simulink model "arducopter"  (R2021a)
settings: Solver=FixedStepAuto  StartTime=0.0  StopTime=sim.param.timeEnd  FixedStep=sim.param.dt  RelTol=1e-3
undefined symbols (not defined in the file or in its folder): DiscIntNeverNeededParam, sim
libraries: simulink x34, slident x4, vrlib x1
(part 3 of 8)

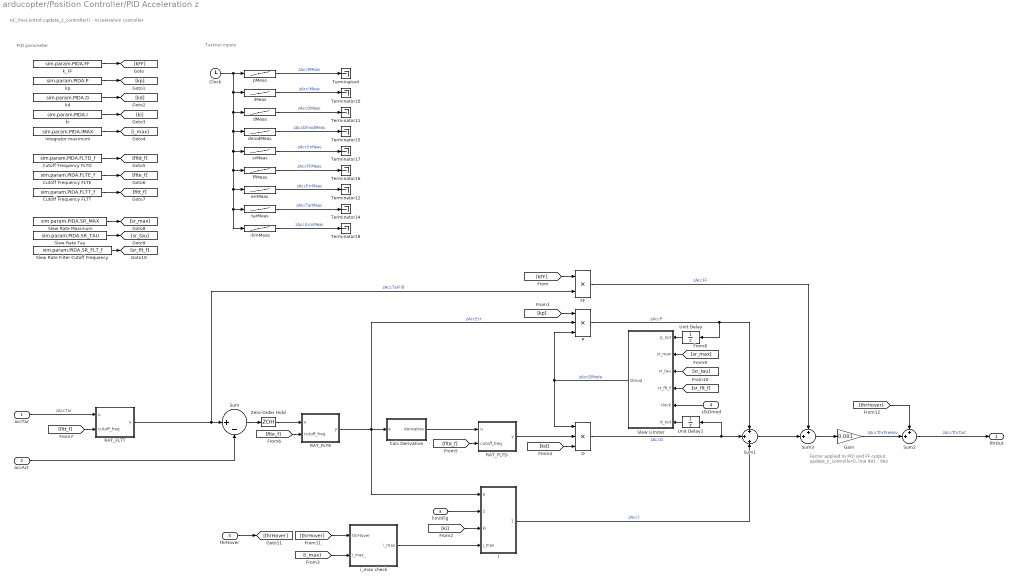
== system arducopter/Position Controller/PID Acceleration z ==
  note: Factor applied to PID and FF output.
      | update_z_controller(), line 991 - 992
  note: AC_PosControl::update_z_controller() - Acceleration controller
  note: PID parameter
  note: Testrun inputs
  accTar : Inport
  accAct : Inport  Port=2
  limitFlg : Inport  Port=3
  clkDmod : Inport  Port=4
  thrHover : Inport  Port=5
  Calc Derivative : Subsystem
  Clock : Clock
  Cutoff Frequency FLTD : Constant  Value=sim.param.PIDA.FLTD_f
  Cutoff Frequency FLTE : Constant  Value=sim.param.PIDA.FLTE_f
  Cutoff Frequency FLTT : Constant  Value=sim.param.PIDA.FLTT_f
  D : Product  Inputs=3
  FF : Product
  Gain : Gain  Gain=0.001
  I : Subsystem
  Integrator maximum : Constant  Value=sim.param.PIDA.IMAX
  P : Product  Inputs=3
  RAT_FLTD : Subsystem  TreatAsAtomicUnit=on  SystemSampleTime=sim.param.dt
  RAT_FLTE : Subsystem  TreatAsAtomicUnit=on  SystemSampleTime=sim.param.dt
  RAT_FLTT : Subsystem  TreatAsAtomicUnit=on  SystemSampleTime=sim.param.dt
  Slew Limiter : Subsystem
  Slew Rate Filter Cutoff Frequency : Constant  Value=sim.param.PIDA.SR_FLT_f
  Slew Rate Maximum : Constant  Value=sim.param.PIDA.SR_MAX
  Slew Rate Tau : Constant  Value=sim.param.PIDA.SR_TAU
  Sum : Sum  Inputs=|+-
  Sum1 : Sum  Inputs=+|+|+
  Sum2 : Sum  Inputs=++|  OutDataTypeStr=single
  Sum3 : Sum  Inputs=++|  OutDataTypeStr=single
  Terminator{4,10..12,14..18} (9 alike) : Terminator
  Unit Delay : UnitDelay  InitialCondition=sim.init.PIDA.P  SampleTime=-1  HasFrameUpgradeWarning=on
  Unit Delay1 : UnitDelay  InitialCondition=sim.init.PIDA.D  SampleTime=-1  HasFrameUpgradeWarning=on
  Zero-Order Hold : ZeroOrderHold  SampleTime=-1
  dMeas : Lookup_n-D  NumberOfTableDimensions=1  BreakpointsForDimension1=sim.signals.PIDR.Time  Table=sim.signals.PIDR.D  InternalRulePriority=Speed  RndMeth=Simplest  InputSameDT=on
  dmodMeas : Lookup_n-D  NumberOfTableDimensions=1  BreakpointsForDimension1=sim.signals.PIDA.Time  Table=sim.signals.PIDA.DMod  InternalRulePriority=Speed  RndMeth=Simplest  InputSameDT=on
  errMeas : Lookup_n-D  NumberOfTableDimensions=1  BreakpointsForDimension1=sim.signals.PIDA.Time  Table=sim.signals.PIDA.Err  InternalRulePriority=Speed  RndMeth=Simplest  InputSameDT=on
  ffMeas : Lookup_n-D  NumberOfTableDimensions=1  BreakpointsForDimension1=sim.signals.PIDA.Time  Table=sim.signals.PIDA.FF  InternalRulePriority=Speed  RndMeth=Simplest  InputSameDT=on
  iMeas : Lookup_n-D  NumberOfTableDimensions=1  BreakpointsForDimension1=sim.signals.PIDA.Time  Table=sim.signals.PIDA.I  InternalRulePriority=Speed  RndMeth=Simplest  InputSameDT=on
  i_max check : Subsystem
  ilimMeas : Lookup_n-D  NumberOfTableDimensions=1  BreakpointsForDimension1=sim.signals.PIDA.Time  Table=sim.signals.PIDA.ILimit  InternalRulePriority=Speed  RndMeth=Simplest  InputSameDT=on
  k_FF : Constant  Value=sim.param.PIDA.FF
  kd : Constant  Value=sim.param.PIDA.D
  ki : Constant  Value=sim.param.PIDA.I
  kp : Constant  Value=sim.param.PIDA.P
  pMeas : Lookup_n-D  NumberOfTableDimensions=1  BreakpointsForDimension1=sim.signals.PIDA.Time  Table=sim.signals.PIDA.P  InternalRulePriority=Speed  RndMeth=Simplest  InputSameDT=on
  srMeas : Lookup_n-D  NumberOfTableDimensions=1  BreakpointsForDimension1=sim.signals.PIDA.Time  Table=sim.signals.PIDA.SRate  InternalRulePriority=Speed  RndMeth=Simplest  InputSameDT=on
  tarMeas : Lookup_n-D  NumberOfTableDimensions=1  BreakpointsForDimension1=sim.signals.PIDA.Time  Table=sim.signals.PIDA.Tar  InternalRulePriority=Speed  RndMeth=Simplest  InputSameDT=on
  thrOut : Outport
  wires:
  RAT_FLTD/1(y) -> D/2
  Sum1/1 -> Sum3/2
  limitFlg/1 -> I/2(limitFlg)
  P/1 -> Unit Delay/1, Sum1/1  "zAccP"
  Calc Derivative/1(derivative) -> RAT_FLTD/1(u)
  Sum/1 -> Zero-Order Hold/1
  D/1 -> Unit Delay1/1, Sum1/2  "zAccD"
  I/1(integrator) -> Sum1/3  "zAccI"
  FF/1 -> Sum3/1  "zAccFF"
  Sum3/1 -> Gain/1
  RAT_FLTT/1(y) -> FF/2, Sum/1  "zAccTarFilt"
  Zero-Order Hold/1 -> RAT_FLTE/1(u)
  k_FF/1 -> [kFF]
  kp/1 -> [kp]
  kd/1 -> [kd]
  ki/1 -> [ki]
  Integrator maximum/1 -> [i_max]
  Cutoff Frequency FLTD/1 -> [fltd_f]
  Cutoff Frequency FLTE/1 -> [flte_f]
  Cutoff Frequency FLTT/1 -> [fltt_f]
  [kFF] -> FF/1
  [kp] -> P/1
  [ki] -> I/3(ki)
  [kd] -> D/3
  [fltd_f] -> RAT_FLTD/2(cutoff_freq)
  [flte_f] -> RAT_FLTE/2(cutoff_freq)
  [fltt_f] -> RAT_FLTT/2(cutoff_freq)
  RAT_FLTE/1(y) -> P/2, Calc Derivative/1(e), I/1(e)  "zAccErr"
  Slew Rate Filter Cutoff Frequency/1 -> [sr_flt_f]
  Slew Rate Maximum/1 -> [sr_max]
  Slew Rate Tau/1 -> [sr_tau]
  Slew Limiter/1(Dmod) -> D/1, P/3  "zAccDMode"
  Unit Delay/1 -> Slew Limiter/1(p_out)
  Unit Delay1/1 -> Slew Limiter/6(d_out)
  [sr_max] -> Slew Limiter/2(sr_max)
  [sr_tau] -> Slew Limiter/3(sr_tau)
  [sr_flt_f] -> Slew Limiter/4(sr_flt_f)
  clkDmod/1 -> Slew Limiter/5(clock)
  [thrHover] -> i_max check/1(thrHover)
  [i_max] -> i_max check/2(i_max_)
  i_max check/1(i_max) -> I/4(i_max)
  Sum2/1 -> thrOut/1  "zAccThrOut"
  thrHover/1 -> [thrHover]
  Gain/1 -> Sum2/2  "zAccThrPreHov"
  [thrHover] -> Sum2/1
  Clock/1 -> ilimMeas/1, tarMeas/1, errMeas/1, ffMeas/1, srMeas/1, dmodMeas/1, dMeas/1, iMeas/1, pMeas/1
  dmodMeas/1 -> Terminator15/1  "zAccDmodMeas"
  ilimMeas/1 -> Terminator18/1  "zAccILimMeas"
  srMeas/1 -> Terminator17/1  "zAccSrMeas"
  iMeas/1 -> Terminator10/1  "zAccIMeas"
  ffMeas/1 -> Terminator16/1  "zAccFFMeas"
  pMeas/1 -> Terminator4/1  "zAccPMeas"
  errMeas/1 -> Terminator12/1  "zAccErrMeas"
  tarMeas/1 -> Terminator14/1  "zAccTarMeas"
  dMeas/1 -> Terminator11/1  "zAccDMeas"
  accAct/1 -> Sum/2
  accTar/1 -> RAT_FLTT/1(u)  "zAccTar"

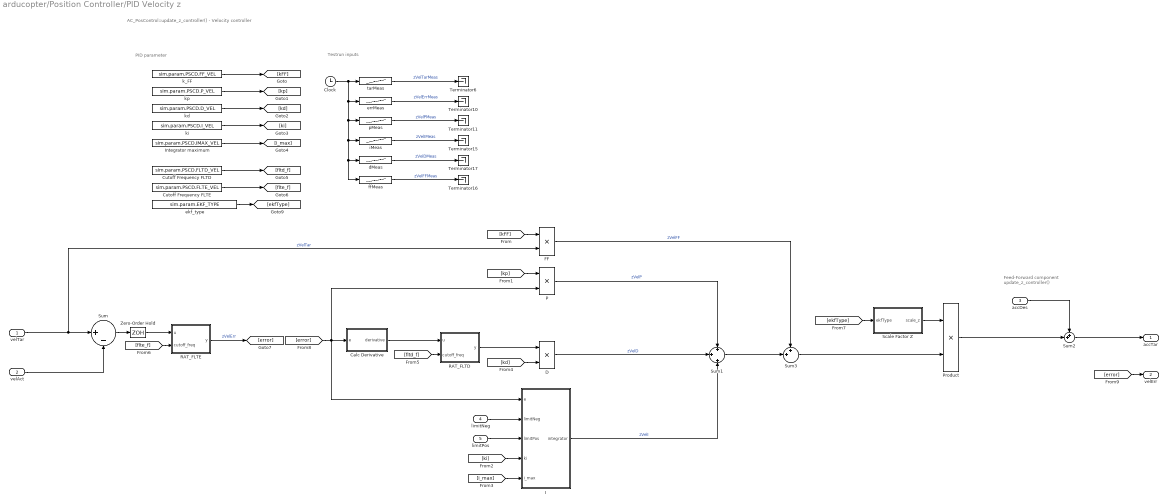
== system arducopter/Position Controller/PID Velocity z ==
  note: PID parameter
  note: Testrun inputs
  note: Feed-Forward component
      | update_z_controller()
  note: AC_PosControl::update_z_controller() - Velocity controller
  velTar : Inport
  velAct : Inport  Port=2
  accDes : Inport  Port=3
  limitNeg : Inport  Port=4
  limitPos : Inport  Port=5
  Calc Derivative : Subsystem
  Clock : Clock
  Cutoff Frequency FLTD : Constant  Value=sim.param.PSCD.FLTD_VEL
  Cutoff Frequency FLTE : Constant  Value=sim.param.PSCD.FLTE_VEL
  D : Product
  FF : Product
  I : Subsystem
  Integrator maximum : Constant  Value=sim.param.PSCD.IMAX_VEL
  P : Product
  Product : Product
  RAT_FLTD : Subsystem  TreatAsAtomicUnit=on  SystemSampleTime=sim.param.dt
  RAT_FLTE : Subsystem  TreatAsAtomicUnit=on  SystemSampleTime=sim.param.dt
  Scale Factor Z : Subsystem
  Sum : Sum  Inputs=|+-
  Sum1 : Sum  Inputs=+|+|+
  Sum2 : Sum  Inputs=++|
  Sum3 : Sum  Inputs=++|  OutDataTypeStr=single
  Terminator{6,10..11,15..17} (6 alike) : Terminator
  Zero-Order Hold : ZeroOrderHold  SampleTime=-1
  dMeas : Lookup_n-D  NumberOfTableDimensions=1  BreakpointsForDimension1=sim.signals.PCVZ.Time  Table=sim.signals.PCVZ.D  InternalRulePriority=Speed  RndMeth=Simplest  InputSameDT=on
  ekf_type : Constant  Value=sim.param.EKF_TYPE
  errMeas : Lookup_n-D  NumberOfTableDimensions=1  BreakpointsForDimension1=sim.signals.PCVZ.Time  Table=sim.signals.PCVZ.Err  InternalRulePriority=Speed  RndMeth=Simplest  InputSameDT=on
  ffMeas : Lookup_n-D  NumberOfTableDimensions=1  BreakpointsForDimension1=sim.signals.PCVZ.Time  Table=sim.signals.PCVZ.FF  InternalRulePriority=Speed  RndMeth=Simplest  InputSameDT=on
  iMeas : Lookup_n-D  NumberOfTableDimensions=1  BreakpointsForDimension1=sim.signals.PCVZ.Time  Table=sim.signals.PCVZ.I  InternalRulePriority=Speed  RndMeth=Simplest  InputSameDT=on
  k_FF : Constant  Value=sim.param.PSCD.FF_VEL
  kd : Constant  Value=sim.param.PSCD.D_VEL
  ki : Constant  Value=sim.param.PSCD.I_VEL
  kp : Constant  Value=sim.param.PSCD.P_VEL
  pMeas : Lookup_n-D  NumberOfTableDimensions=1  BreakpointsForDimension1=sim.signals.PCVZ.Time  Table=sim.signals.PCVZ.P  InternalRulePriority=Speed  RndMeth=Simplest  InputSameDT=on
  tarMeas : Lookup_n-D  NumberOfTableDimensions=1  BreakpointsForDimension1=sim.signals.PSCD.Time  Table=sim.signals.PSCD.zVelTar  InternalRulePriority=Speed  RndMeth=Simplest  InputSameDT=on
  accTar : Outport
  velErr : Outport  Port=2
  wires:
  RAT_FLTD/1(y) -> D/1
  Sum1/1 -> Sum3/2
  [error] -> I/1(e), P/2, Calc Derivative/1(e)
  limitNeg/1 -> I/2(limitNeg)
  P/1 -> Sum1/1  "zVelP"
  Calc Derivative/1(derivative) -> RAT_FLTD/1(u)
  Sum/1 -> Zero-Order Hold/1
  D/1 -> Sum1/2  "zVelD"
  I/1(integrator) -> Sum1/3  "zVelI"
  FF/1 -> Sum3/1  "zVelFF"
  velAct/1 -> Sum/2
  Zero-Order Hold/1 -> RAT_FLTE/1(u)
  k_FF/1 -> [kFF]
  kp/1 -> [kp]
  kd/1 -> [kd]
  ki/1 -> [ki]
  Integrator maximum/1 -> [i_max]
  Cutoff Frequency FLTD/1 -> [fltd_f]
  Cutoff Frequency FLTE/1 -> [flte_f]
  [kFF] -> FF/1
  [kp] -> P/1
  [ki] -> I/4(ki)
  [i_max] -> I/5(i_max)
  [kd] -> D/2
  [fltd_f] -> RAT_FLTD/2(cutoff_freq)
  [flte_f] -> RAT_FLTE/2(cutoff_freq)
  velTar/1 -> FF/2, Sum/1  "zVelTar"
  limitPos/1 -> I/3(limitPos)
  Sum3/1 -> Product/2
  [ekfType] -> Scale Factor Z/1(ekfType)
  Scale Factor Z/1(scale_z) -> Product/1
  accDes/1 -> Sum2/1
  Sum2/1 -> accTar/1
  Product/1 -> Sum2/2
  ekf_type/1 -> [ekfType]
  RAT_FLTE/1(y) -> [error]  "zVelErr"
  [error] -> velErr/1
  Clock/1 -> ffMeas/1, dMeas/1, iMeas/1, pMeas/1, errMeas/1, tarMeas/1
  tarMeas/1 -> Terminator6/1  "zVelTarMeas"
  pMeas/1 -> Terminator11/1  "zVelPMeas"
  ffMeas/1 -> Terminator16/1  "zVelFFMeas"
  dMeas/1 -> Terminator17/1  "zVelDMeas"
  iMeas/1 -> Terminator15/1  "zVelIMeas"
  errMeas/1 -> Terminator10/1  "zVelErrMeas"

== system arducopter/Position Controller/calc des climb rate ==
  note: Constrain target_climb_rate
  note: Calculation of desired climb rate from throttle control input.
      | Based on ModeAltHold::run(), where Copter::get_pilot_desired_climb_rate() is called from
  ctrlIn : Inport
  Constant1 : Constant  Value=sim.param.PSCD.VEL_MAX_DN
  Constant18 : Constant  Value=sim.param.PSCD.THR_DZ
  Constant19 : Constant  Value=sim.param.RCIN.MIN_THR
  Constant2 : Constant  Value=sim.param.PSCD.VEL_MAX_UP
  Constant20 : Constant  Value=sim.param.RCIN.MAX_THR
  Constant21 : Constant  Value=sim.param.RCIN.REVERSED_THR
  Constant22 : Constant  Value=1000
  Constant3 : Constant  Value=sim.param.RCIN.DZ_THR
  MATLAB Function : MATLAB Function  TreatAsAtomicUnit=on
  contrain climb rate : Subsystem
  climbRate : Outport
  wires:
  ctrlIn/1 -> MATLAB Function/1(ctrlIn)
  MATLAB Function/1(climbRateDes) -> contrain climb rate/1(in)
  Constant18/1 -> MATLAB Function/2(deadZoneThr)
  Constant19/1 -> MATLAB Function/4(radioMin)
  Constant20/1 -> MATLAB Function/5(radioMax)
  Constant21/1 -> MATLAB Function/6(reversed)
  Constant22/1 -> MATLAB Function/7(highIn)
  Constant1/1 -> MATLAB Function/8(maxSpeedDn)
  Constant2/1 -> MATLAB Function/9(maxSpeedUp)
  contrain climb rate/1(out) -> climbRate/1
  Constant3/1 -> MATLAB Function/3(deadZoneRC)

== system arducopter/Position Controller/get_pilot_speed_dn() ==
  upMax : Inport
  MATLAB Function : MATLAB Function  TreatAsAtomicUnit=on
  dnSpeedMax : Constant  Value=sim.param.PSCD.VEL_MAX_DN
  dnMax : Outport
  wires:
  dnSpeedMax/1 -> MATLAB Function/1(dnMaxIn)
  upMax/1 -> MATLAB Function/2(upMax)
  MATLAB Function/1(dnMax) -> dnMax/1

== system arducopter/Position Controller/input handler ==
  inSim : Inport
  inMeas : Inport  Port=2
  Constant : Constant  Value=sim.param.mdlVal
  Switch : Switch  Criteria=u2 > Threshold
  inAct : Outport
  wires:
  inSim/1 -> Switch/1
  inMeas/1 -> Switch/3
  Switch/1 -> inAct/1
  Constant/1 -> Switch/2

== system arducopter/Position Controller/set z component of limit vec ==
  note: Set vertical component of limit vector based on throttle limits of motors
  limitLower : Inport
  limitUpper : Inport  Port=2
  MATLAB Function : MATLAB Function  TreatAsAtomicUnit=on
  limitVectorZ : Outport
  wires:
  limitLower/1 -> MATLAB Function/1(limLower)
  limitUpper/1 -> MATLAB Function/2(limUpper)
  MATLAB Function/1(limVecZ) -> limitVectorZ/1

== system arducopter/Position Controller/set_pos_target_z_from_climb_rate() ==
  note: input_vel_accel_z()
      | Calculate a jerk limited path from the current position, velocity and acceleration to an input acceleration
  note: set_pos_target_z_from_climb_rate
      | Calculation of target position and desired vel. and accel
  posTarIn : Inport
  climbRateDes : Inport  Port=2
  limitVectorZ : Inport  Port=3
  velMaxUp : Inport  Port=4
  velMaxDn : Inport  Port=5
  accMaxZ : Inport  Port=6
  jerkMaxZ : Inport  Port=7
  posErr : Inport  Port=8
  velErr : Inport  Port=9
  Constant : Constant  Value=0  OutDataTypeStr=single
  Data Store Memory : DataStoreMemory  DataStoreName=velDes  ReadBeforeWriteMsg=warning  WriteAfterWriteMsg=warning  WriteAfterReadMsg=warning  InitialValue=sim.init.PIDA.velDes  ShowAdditionalParam=off  OutDataTypeStr=single
  Data Store Memory1 : DataStoreMemory  DataStoreName=accDes  ReadBeforeWriteMsg=warning  WriteAfterWriteMsg=warning  WriteAfterReadMsg=warning  InitialValue=sim.init.PIDA.accDes  ShowAdditionalParam=off  OutDataTypeStr=single
  Data Store Read : DataStoreRead  DataStoreName=velDes  IndexOptions=Index vector (dialog)  Indices=1  OutputSizes=1
  Data Store Read1 : DataStoreRead  DataStoreName=accDes  IndexOptions=Index vector (dialog)  Indices=1  OutputSizes=1
  Data Store Read4 : DataStoreRead  DataStoreName=velDes  IndexOptions=Index vector (dialog)  Indices=1  OutputSizes=1
  Data Store Read5 : DataStoreRead  DataStoreName=accDes  IndexOptions=Index vector (dialog)  Indices=1  OutputSizes=1
  Data Store Write1 : DataStoreWrite  DataStoreName=velDes  IndexOptions=Index vector (dialog)  Indices=1  OutputSizes=1
  Data Store Write2 : DataStoreWrite  DataStoreName=accDes  IndexOptions=Index vector (dialog)  Indices=1  OutputSizes=1
  input_vel_accel_z : Subsystem
  posTar : Outport
  velDes : Outport  Port=2
  accDes : Outport  Port=3
  wires:
  climbRateDes/1 -> input_vel_accel_z/1(velDesTar)
  velMaxUp/1 -> input_vel_accel_z/4(velMaxUp)
  velMaxDn/1 -> input_vel_accel_z/5(velMaxDn)
  accMaxZ/1 -> input_vel_accel_z/6(accMaxZ)
  Constant/1 -> input_vel_accel_z/2(accDesTar)
  jerkMaxZ/1 -> input_vel_accel_z/7(jerkMax)
  limitVectorZ/1 -> input_vel_accel_z/3(limitVectorZ)
  input_vel_accel_z/2(velDes) -> Data Store Write1/1
  input_vel_accel_z/3(accDes) -> Data Store Write2/1
  input_vel_accel_z/1(posTar) -> posTar/1
  Data Store Read4/1 -> velDes/1
  Data Store Read5/1 -> accDes/1
  posTarIn/1 -> input_vel_accel_z/8(posTarIn)
  Data Store Read/1 -> input_vel_accel_z/11(velDesIn)
  Data Store Read1/1 -> input_vel_accel_z/12(accDesIn)
  velErr/1 -> input_vel_accel_z/10(velErr)
  posErr/1 -> input_vel_accel_z/9(posErr)

== system arducopter/Position Controller/zVelCtrlRatio Calculation ==
  note: Update vel_z_control_ratio
      | AC_PosControl.cpp, update_z_controller()
  velErr : Inport
  dnVelMax : Inport  Port=2
  Constant1 : Constant  Value=sim.param.dt
  Data Store Memory : DataStoreMemory  DataStoreName=vel_z_ctrl_ratio  ReadBeforeWriteMsg=warning  WriteAfterWriteMsg=warning  WriteAfterReadMsg=warning  InitialValue=sim.param.PSCD.CTRL_RATIO_INIT  ShowAdditionalParam=off  OutDataTypeStr=single
  Data Type Conversion1 : DataTypeConversion  OutDataTypeStr=single
  Update vel_z_ctrl_ratio : MATLAB Function  TreatAsAtomicUnit=on
  zVelCtrlRatio : Outport
  wires:
  Constant1/1 -> Data Type Conversion1/1
  velErr/1 -> Update vel_z_ctrl_ratio/1(velErr)
  dnVelMax/1 -> Update vel_z_ctrl_ratio/2(dnVelMax)
  Data Type Conversion1/1 -> Update vel_z_ctrl_ratio/3(dt)
  Update vel_z_ctrl_ratio/1(zVelCtrlRat) -> zVelCtrlRatio/1

== system arducopter/Rate Controller/Input Handler ==
  note: Actual Values
  note: Desired Values
  note: Use measured desired values for rate controller validation
  note: Use measured actual values for rate controller validation
  inMeas : Inport
  inSim : Inport  Port=2
  Bus Creator : BusCreator  Inputs=6
  Bus Selector : BusSelector  OutputSignals=RATE.rollRateTarMeas,RATE.pitchRateTarMeas,RATE.yawRateTarMeas
  Bus Selector1 : BusSelector  OutputSignals=rollRateTar,pitchRateTar,yawRateTar
  Bus Selector2 : BusSelector  OutputSignals=PIDR.rollRateActMeas,PIDP.pitchRateActMeas,PIDY.yawRateActMeas
  Bus Selector3 : BusSelector  OutputSignals=rollRateAct,pitchRateAct,yawRateAct
  Constant1 : Constant  Value=sim.param.attCtrlVal
  Constant2 : Constant  Value=sim.param.attCtrlVal
  Constant3 : Constant  Value=sim.param.rateCtrlVal
  Constant4 : Constant  Value=sim.param.rateCtrlVal
  Demux : Demux  Outputs=3
  Demux1 : Demux  Outputs=3
  OR : Logic  Operator=OR  AllPortsSameDT=off  OutDataTypeStr=boolean
  OR1 : Logic  Operator=OR  AllPortsSameDT=off  OutDataTypeStr=boolean
  Switch : Switch  Criteria=u2 > Threshold
  Switch1 : Switch  Criteria=u2 > Threshold
  Vector Concatenate{,1..3} (4 alike) : Concatenate  NumInputs=3
  in : Outport
  wires:
  Bus Creator/1 -> in/1
  inMeas/1 -> Bus Selector2/1, Bus Selector/1
  Bus Selector/1 -> Vector Concatenate/1  "<rollRateTarMeas>"
  Bus Selector/2 -> Vector Concatenate/2  "<pitchRateTarMeas>"
  Bus Selector/3 -> Vector Concatenate/3  "<yawRateTarMeas>"
  inSim/1 -> Bus Selector1/1, Bus Selector3/1
  Bus Selector1/1 -> Vector Concatenate1/1  "<rollRateTar>"
  Bus Selector1/2 -> Vector Concatenate1/2  "<pitchRateTar>"
  Bus Selector1/3 -> Vector Concatenate1/3  "<yawRateTar>"
  Vector Concatenate/1 -> Switch/1
  Vector Concatenate1/1 -> Switch/3
  Bus Selector2/1 -> Vector Concatenate2/1  "<rollRateActMeas>"
  Bus Selector2/2 -> Vector Concatenate2/2  "<pitchRateActMeas>"
  Bus Selector2/3 -> Vector Concatenate2/3  "<yawRateActMeas>"
  Vector Concatenate2/1 -> Switch1/1
  Bus Selector3/1 -> Vector Concatenate3/1  "<rollRateAct>"
  Bus Selector3/2 -> Vector Concatenate3/2  "<pitchRateAct>"
  Bus Selector3/3 -> Vector Concatenate3/3  "<yawRateAct>"
  Vector Concatenate3/1 -> Switch1/3
  Switch/1 -> Demux/1
  Switch1/1 -> Demux1/1
  Demux1/1 -> Bus Creator/4  "rollRateAct"
  Demux1/2 -> Bus Creator/5  "pitchRateAct"
  Demux1/3 -> Bus Creator/6  "yawRateAct"
  Demux/1 -> Bus Creator/1  "rollRateTar"
  Demux/2 -> Bus Creator/2  "pitchRateTar"
  Demux/3 -> Bus Creator/3  "yawRateTar"
  OR/1 -> Switch/2
  Constant4/1 -> OR/1
  Constant1/1 -> OR/2
  Constant2/1 -> OR1/2
  Constant3/1 -> OR1/1
  OR1/1 -> Switch1/2

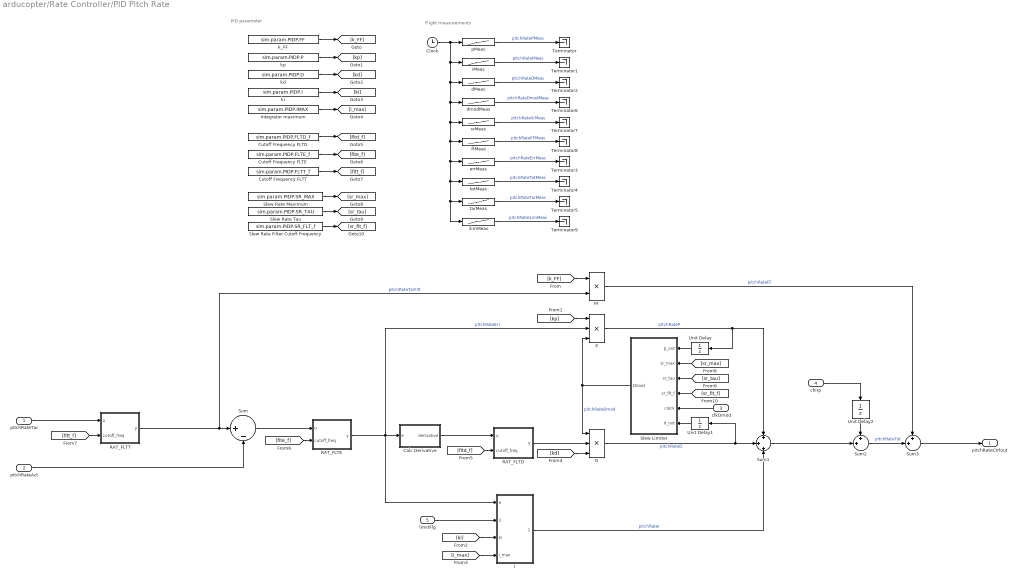
== system arducopter/Rate Controller/PID Pitch Rate ==
  note: PID parameter
  note: Flight measurements
  pitchRateTar : Inport
  pitchRateAct : Inport  Port=2
  clkDmod : Inport  Port=3
  chirp : Inport  Port=4
  limitFlg : Inport  Port=5
  Calc Derivative : Subsystem
  Clock : Clock
  Cutoff Frequency FLTD : Constant  Value=sim.param.PIDP.FLTD_f
  Cutoff Frequency FLTE : Constant  Value=sim.param.PIDP.FLTE_f
  Cutoff Frequency FLTT : Constant  Value=sim.param.PIDP.FLTT_f
  D : Product  Inputs=3
  FF : Product
  I : Subsystem
  Integrator maximum : Constant  Value=sim.param.PIDP.IMAX
  P : Product  Inputs=3
  RAT_FLTD : Subsystem  TreatAsAtomicUnit=on  SystemSampleTime=sim.param.dt
  RAT_FLTE : Subsystem  TreatAsAtomicUnit=on  SystemSampleTime=sim.param.dt
  RAT_FLTT : Subsystem  TreatAsAtomicUnit=on  SystemSampleTime=sim.param.dt
  Slew Limiter : Subsystem
  Slew Rate Filter Cutoff Frequency : Constant  Value=sim.param.PIDP.SR_FLT_f
  Slew Rate Maximum : Constant  Value=sim.param.PIDP.SR_MAX
  Slew Rate Tau : Constant  Value=sim.param.PIDP.SR_TAU
  Sum : Sum  Inputs=|+-
  Sum1 : Sum  Inputs=+|+|+
  Sum2 : Sum  Inputs=++|
  Sum3 : Sum  Inputs=++|  OutDataTypeStr=single
  Terminator{,1..9} (10 alike) : Terminator
  Unit Delay : UnitDelay  InitialCondition=sim.init.PIDP.P  SampleTime=-1  HasFrameUpgradeWarning=on
  Unit Delay1 : UnitDelay  InitialCondition=sim.init.PIDP.D  SampleTime=-1  HasFrameUpgradeWarning=on
  Unit Delay2 : UnitDelay  SampleTime=-1  HasFrameUpgradeWarning=on
  dMeas : Lookup_n-D  NumberOfTableDimensions=1  BreakpointsForDimension1=sim.signals.PIDP.Time  Table=sim.signals.PIDP.D  InternalRulePriority=Speed  RndMeth=Simplest  InputSameDT=on
  dmodMeas : Lookup_n-D  NumberOfTableDimensions=1  BreakpointsForDimension1=sim.signals.PIDP.Time  Table=sim.signals.PIDP.DMod  InternalRulePriority=Speed  RndMeth=Simplest  InputSameDT=on
  errMeas : Lookup_n-D  NumberOfTableDimensions=1  BreakpointsForDimension1=sim.signals.PIDP.Time  Table=sim.signals.PIDP.Err  InternalRulePriority=Speed  RndMeth=Simplest  InputSameDT=on
  ffMeas : Lookup_n-D  NumberOfTableDimensions=1  BreakpointsForDimension1=sim.signals.PIDP.Time  Table=sim.signals.PIDP.FF  InternalRulePriority=Speed  RndMeth=Simplest  InputSameDT=on
  iMeas : Lookup_n-D  NumberOfTableDimensions=1  BreakpointsForDimension1=sim.signals.PIDP.Time  Table=sim.signals.PIDP.I  InternalRulePriority=Speed  RndMeth=Simplest  InputSameDT=on
  ilimMeas : Lookup_n-D  NumberOfTableDimensions=1  BreakpointsForDimension1=sim.signals.PIDP.Time  Table=sim.signals.PIDP.ILimit  InternalRulePriority=Speed  RndMeth=Simplest  InputSameDT=on
  k_FF : Constant  Value=sim.param.PIDP.FF
  kd : Constant  Value=sim.param.PIDP.D
  ki : Constant  Value=sim.param.PIDP.I
  kp : Constant  Value=sim.param.PIDP.P
  pMeas : Lookup_n-D  NumberOfTableDimensions=1  BreakpointsForDimension1=sim.signals.PIDP.Time  Table=sim.signals.PIDP.P  InternalRulePriority=Speed  RndMeth=Simplest  InputSameDT=on
  srMeas : Lookup_n-D  NumberOfTableDimensions=1  BreakpointsForDimension1=sim.signals.PIDP.Time  Table=sim.signals.PIDP.SRate  InternalRulePriority=Speed  RndMeth=Simplest  InputSameDT=on
  tarMeas : Lookup_n-D  NumberOfTableDimensions=1  BreakpointsForDimension1=sim.signals.PIDP.Time  Table=sim.signals.PIDP.Tar  InternalRulePriority=Speed  RndMeth=Simplest  InputSameDT=on
  totMeas : Lookup_n-D  NumberOfTableDimensions=1  BreakpointsForDimension1=sim.signals.RATE.Time  Table=sim.signals.RATE.POut  InternalRulePriority=Speed  RndMeth=Simplest  InputSameDT=on
  pitchRateCtrlout : Outport
  wires:
  [flte_f] -> RAT_FLTE/2(cutoff_freq)
  Cutoff Frequency FLTT/1 -> [fltt_f]
  Cutoff Frequency FLTE/1 -> [flte_f]
  Cutoff Frequency FLTD/1 -> [fltd_f]
  Integrator maximum/1 -> [i_max]
  ki/1 -> [ki]
  kd/1 -> [kd]
  kp/1 -> [kp]
  k_FF/1 -> [k_FF]
  Sum/1 -> RAT_FLTE/1(u)
  pitchRateAct/1 -> Sum/2
  chirp/1 -> Unit Delay2/1
  pitchRateTar/1 -> RAT_FLTT/1(u)
  RAT_FLTT/1(y) -> Sum/1, FF/2  "pitchRateTarFilt"
  Sum2/1 -> Sum3/2  "pitchRateTot"
  I/1(integrator) -> Sum1/3  "pitchRateI"
  D/1 -> Unit Delay1/1, Sum1/2  "pitchRateD"
  Calc Derivative/1(derivative) -> RAT_FLTD/1(u)
  P/1 -> Unit Delay/1, Sum1/1  "pitchRateP"
  limitFlg/1 -> I/2(limit_flg)
  RAT_FLTE/1(y) -> I/1(e), Calc Derivative/1(e), P/2  "pitchRateErr"
  RAT_FLTD/1(y) -> D/2
  pMeas/1 -> Terminator/1  "pitchRatePMeas"
  iMeas/1 -> Terminator1/1  "pitchRateIMeas"
  dMeas/1 -> Terminator2/1  "pitchRateDMeas"
  totMeas/1 -> Terminator4/1  "pitchRateTotMeas"
  tarMeas/1 -> Terminator5/1  "pitchRateTarMeas"
  errMeas/1 -> Terminator3/1  "pitchRateErrMeas"
  Slew Limiter/1(Dmod) -> D/1, P/3  "pitchRateDmod"
  Unit Delay/1 -> Slew Limiter/1(p_out)
  Unit Delay1/1 -> Slew Limiter/6(d_out)
  dmodMeas/1 -> Terminator6/1  "pitchRateDmodMeas"
  srMeas/1 -> Terminator7/1  "pitchRateSrMeas"
  ffMeas/1 -> Terminator8/1  "pitchRateFFMeas"
  Slew Rate Maximum/1 -> [sr_max]
  Slew Rate Tau/1 -> [sr_tau]
  Slew Rate Filter Cutoff Frequency/1 -> [sr_flt_f]
  [sr_max] -> Slew Limiter/2(sr_max)
  [sr_tau] -> Slew Limiter/3(sr_tau)
  [sr_flt_f] -> Slew Limiter/4(sr_flt_f)
  ilimMeas/1 -> Terminator9/1  "pitchRateILimMeas"
  clkDmod/1 -> Slew Limiter/5(clock)
  FF/1 -> Sum3/1  "pitchRateFF"
  Unit Delay2/1 -> Sum2/1
  Clock/1 -> ilimMeas/1, tarMeas/1, totMeas/1, errMeas/1, ffMeas/1, srMeas/1, dmodMeas/1, dMeas/1, iMeas/1, pMeas/1
  Sum1/1 -> Sum2/2
  [i_max] -> I/4(i_max)
  [fltd_f] -> RAT_FLTD/2(cutoff_freq)
  [k_FF] -> FF/1
  [kp] -> P/1
  [kd] -> D/3
  [ki] -> I/3(ki)
  [fltt_f] -> RAT_FLTT/2(cutoff_freq)
  Sum3/1 -> pitchRateCtrlout/1

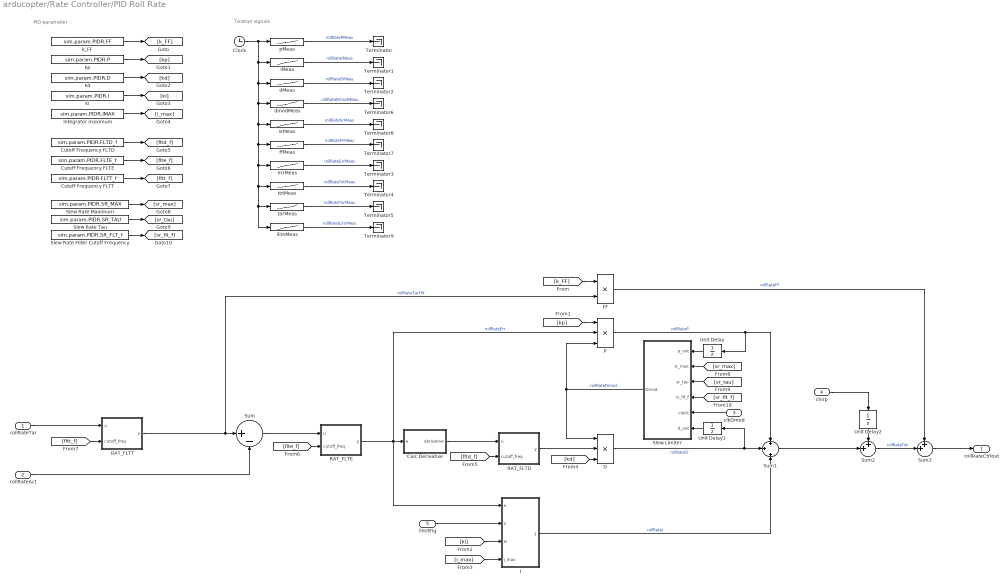
== system arducopter/Rate Controller/PID Roll Rate ==
  note: Testrun signals
  note: PID parameter
  rollRateTar : Inport
  rollRateAct : Inport  Port=2
  clkDmod : Inport  Port=3
  chirp : Inport  Port=4
  limitFlg : Inport  Port=5
  Calc Derivative : Subsystem
  Clock : Clock
  Cutoff Frequency FLTD : Constant  Value=sim.param.PIDR.FLTD_f
  Cutoff Frequency FLTE : Constant  Value=sim.param.PIDR.FLTE_f
  Cutoff Frequency FLTT : Constant  Value=sim.param.PIDR.FLTT_f
  D : Product  Inputs=3
  FF : Product
  I : Subsystem
  Integrator maximum : Constant  Value=sim.param.PIDR.IMAX
  P : Product  Inputs=3
  RAT_FLTD : Subsystem  TreatAsAtomicUnit=on  SystemSampleTime=sim.param.dt
  RAT_FLTE : Subsystem  TreatAsAtomicUnit=on  SystemSampleTime=sim.param.dt
  RAT_FLTT : Subsystem  TreatAsAtomicUnit=on  SystemSampleTime=sim.param.dt
  Slew Limiter : Subsystem
  Slew Rate Filter Cutoff Frequency : Constant  Value=sim.param.PIDR.SR_FLT_f
  Slew Rate Maximum : Constant  Value=sim.param.PIDR.SR_MAX
  Slew Rate Tau : Constant  Value=sim.param.PIDR.SR_TAU
  Sum : Sum  Inputs=|+-
  Sum1 : Sum  Inputs=+|+|+
  Sum2 : Sum  Inputs=++|
  Sum3 : Sum  Inputs=++|  OutDataTypeStr=single
  Terminator{,1..9} (10 alike) : Terminator
  Unit Delay : UnitDelay  InitialCondition=sim.init.PIDR.P  SampleTime=-1  HasFrameUpgradeWarning=on
  Unit Delay1 : UnitDelay  InitialCondition=sim.init.PIDR.D  SampleTime=-1  HasFrameUpgradeWarning=on
  Unit Delay2 : UnitDelay  SampleTime=-1  HasFrameUpgradeWarning=on
  dMeas : Lookup_n-D  NumberOfTableDimensions=1  BreakpointsForDimension1=sim.signals.PIDR.Time  Table=sim.signals.PIDR.D  InternalRulePriority=Speed  RndMeth=Simplest  InputSameDT=on
  dmodMeas : Lookup_n-D  NumberOfTableDimensions=1  BreakpointsForDimension1=sim.signals.PIDR.Time  Table=sim.signals.PIDR.DMod  InternalRulePriority=Speed  RndMeth=Simplest  InputSameDT=on
  errMeas : Lookup_n-D  NumberOfTableDimensions=1  BreakpointsForDimension1=sim.signals.PIDR.Time  Table=sim.signals.PIDR.Err  InternalRulePriority=Speed  RndMeth=Simplest  InputSameDT=on
  ffMeas : Lookup_n-D  NumberOfTableDimensions=1  BreakpointsForDimension1=sim.signals.PIDR.Time  Table=sim.signals.PIDR.FF  InternalRulePriority=Speed  RndMeth=Simplest  InputSameDT=on
  iMeas : Lookup_n-D  NumberOfTableDimensions=1  BreakpointsForDimension1=sim.signals.PIDR.Time  Table=sim.signals.PIDR.I  InternalRulePriority=Speed  RndMeth=Simplest  InputSameDT=on
  ilimMeas : Lookup_n-D  NumberOfTableDimensions=1  BreakpointsForDimension1=sim.signals.PIDR.Time  Table=sim.signals.PIDR.ILimit  InternalRulePriority=Speed  RndMeth=Simplest  InputSameDT=on
  k_FF : Constant  Value=sim.param.PIDR.FF
  kd : Constant  Value=sim.param.PIDR.D
  ki : Constant  Value=sim.param.PIDR.I
  kp : Constant  Value=sim.param.PIDR.P
  pMeas : Lookup_n-D  NumberOfTableDimensions=1  BreakpointsForDimension1=sim.signals.PIDR.Time  Table=sim.signals.PIDR.P  InternalRulePriority=Speed  RndMeth=Simplest  InputSameDT=on
  srMeas : Lookup_n-D  NumberOfTableDimensions=1  BreakpointsForDimension1=sim.signals.PIDR.Time  Table=sim.signals.PIDR.SRate  InternalRulePriority=Speed  RndMeth=Simplest  InputSameDT=on
  tarMeas : Lookup_n-D  NumberOfTableDimensions=1  BreakpointsForDimension1=sim.signals.PIDR.Time  Table=sim.signals.PIDR.Tar  InternalRulePriority=Speed  RndMeth=Simplest  InputSameDT=on
  totMeas : Lookup_n-D  NumberOfTableDimensions=1  BreakpointsForDimension1=sim.signals.RATE.Time  Table=sim.signals.RATE.ROut  InternalRulePriority=Speed  RndMeth=Simplest  InputSameDT=on
  rollRateCtrlout : Outport
  wires:
  RAT_FLTD/1(y) -> D/2
  RAT_FLTE/1(y) -> P/2, Calc Derivative/1(e), I/1(e)  "rollRateErr"
  limitFlg/1 -> I/2(limit_flg)
  P/1 -> Unit Delay/1, Sum1/1  "rollRateP"
  D/1 -> Sum1/2, Unit Delay1/1  "rollRateD"
  I/1(integrator) -> Sum1/3  "rollRateI"
  Sum3/1 -> rollRateCtrlout/1
  RAT_FLTT/1(y) -> FF/2, Sum/1  "rollRateTarFilt"
  rollRateTar/1 -> RAT_FLTT/1(u)
  rollRateAct/1 -> Sum/2
  Sum/1 -> RAT_FLTE/1(u)
  k_FF/1 -> [k_FF]
  kp/1 -> [kp]
  kd/1 -> [kd]
  ki/1 -> [ki]
  Integrator maximum/1 -> [i_max]
  Cutoff Frequency FLTD/1 -> [fltd_f]
  Cutoff Frequency FLTE/1 -> [flte_f]
  Cutoff Frequency FLTT/1 -> [fltt_f]
  [k_FF] -> FF/1
  [kp] -> P/1
  [ki] -> I/3(ki)
  [i_max] -> I/4(i_max)
  [kd] -> D/3
  [fltd_f] -> RAT_FLTD/2(cutoff_freq)
  [flte_f] -> RAT_FLTE/2(cutoff_freq)
  [fltt_f] -> RAT_FLTT/2(cutoff_freq)
  Sum2/1 -> Sum3/2  "rollRateTot"
  pMeas/1 -> Terminator/1  "rollRatePMeas"
  iMeas/1 -> Terminator1/1  "rollRateIMeas"
  errMeas/1 -> Terminator3/1  "rollRateErrMeas"
  dMeas/1 -> Terminator2/1  "rollRateDMeas"
  tarMeas/1 -> Terminator5/1  "rollRateTarMeas"
  totMeas/1 -> Terminator4/1  "rollRateTotMeas"
  Unit Delay/1 -> Slew Limiter/1(p_out)
  Unit Delay1/1 -> Slew Limiter/6(d_out)
  Slew Rate Maximum/1 -> [sr_max]
  [sr_max] -> Slew Limiter/2(sr_max)
  Slew Rate Tau/1 -> [sr_tau]
  Slew Rate Filter Cutoff Frequency/1 -> [sr_flt_f]
  [sr_tau] -> Slew Limiter/3(sr_tau)
  [sr_flt_f] -> Slew Limiter/4(sr_flt_f)
  Slew Limiter/1(Dmod) -> D/1, P/3  "rollRateDmod"
  Sum1/1 -> Sum2/2
  chirp/1 -> Unit Delay2/1
  Unit Delay2/1 -> Sum2/1
  FF/1 -> Sum3/1  "rollRateFF"
  Calc Derivative/1(derivative) -> RAT_FLTD/1(u)
  dmodMeas/1 -> Terminator6/1  "rollRateDmodMeas"
  ffMeas/1 -> Terminator7/1  "rollRateFFMeas"
  srMeas/1 -> Terminator8/1  "rollRateSrMeas"
  clkDmod/1 -> Slew Limiter/5(clock)
  ilimMeas/1 -> Terminator9/1  "rollRateILimMeas"
  Clock/1 -> ilimMeas/1, tarMeas/1, totMeas/1, errMeas/1, ffMeas/1, srMeas/1, dmodMeas/1, dMeas/1, iMeas/1, pMeas/1

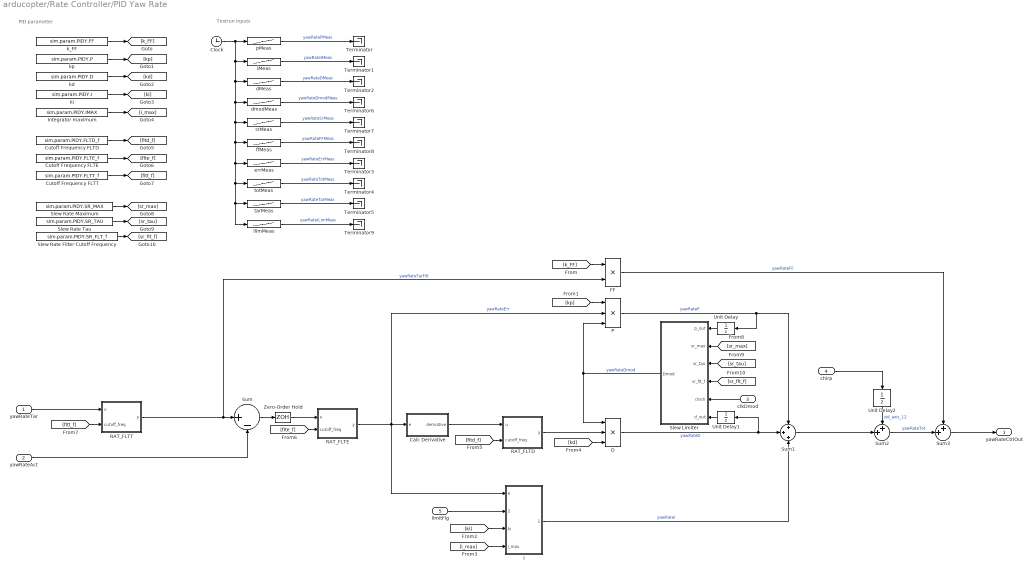
== system arducopter/Rate Controller/PID Yaw Rate ==
  note: PID parameter
  note: Testrun inputs
  yawRateTar : Inport
  yawRateAct : Inport  Port=2
  clkDmod : Inport  Port=3
  chirp : Inport  Port=4
  limitFlg : Inport  Port=5
  Calc Derivative : Subsystem
  Clock : Clock
  Cutoff Frequency FLTD : Constant  Value=sim.param.PIDY.FLTD_f
  Cutoff Frequency FLTE : Constant  Value=sim.param.PIDY.FLTE_f
  Cutoff Frequency FLTT : Constant  Value=sim.param.PIDY.FLTT_f
  D : Product  Inputs=3
  FF : Product
  I : Subsystem
  Integrator maximum : Constant  Value=sim.param.PIDY.IMAX
  P : Product  Inputs=3
  RAT_FLTD : Subsystem  TreatAsAtomicUnit=on  SystemSampleTime=sim.param.dt
  RAT_FLTE : Subsystem  TreatAsAtomicUnit=on  SystemSampleTime=sim.param.dt
  RAT_FLTT : Subsystem  TreatAsAtomicUnit=on  SystemSampleTime=sim.param.dt
  Slew Limiter : Subsystem
  Slew Rate Filter Cutoff Frequency : Constant  Value=sim.param.PIDY.SR_FLT_f
  Slew Rate Maximum : Constant  Value=sim.param.PIDY.SR_MAX
  Slew Rate Tau : Constant  Value=sim.param.PIDY.SR_TAU
  Sum : Sum  Inputs=|+-
  Sum1 : Sum  Inputs=+|+|+
  Sum2 : Sum  Inputs=++|
  Sum3 : Sum  Inputs=++|  OutDataTypeStr=single
  Terminator{,1..9} (10 alike) : Terminator
  Unit Delay : UnitDelay  InitialCondition=sim.init.PIDY.P  SampleTime=-1  HasFrameUpgradeWarning=on
  Unit Delay1 : UnitDelay  InitialCondition=sim.init.PIDY.D  SampleTime=-1  HasFrameUpgradeWarning=on
  Unit Delay2 : UnitDelay  SampleTime=-1  HasFrameUpgradeWarning=on
  Zero-Order Hold : ZeroOrderHold  SampleTime=-1
  dMeas : Lookup_n-D  NumberOfTableDimensions=1  BreakpointsForDimension1=sim.signals.PIDY.Time  Table=sim.signals.PIDY.D  InternalRulePriority=Speed  RndMeth=Simplest  InputSameDT=on
  dmodMeas : Lookup_n-D  NumberOfTableDimensions=1  BreakpointsForDimension1=sim.signals.PIDY.Time  Table=sim.signals.PIDY.DMod  InternalRulePriority=Speed  RndMeth=Simplest  InputSameDT=on
  errMeas : Lookup_n-D  NumberOfTableDimensions=1  BreakpointsForDimension1=sim.signals.PIDY.Time  Table=sim.signals.PIDY.Err  InternalRulePriority=Speed  RndMeth=Simplest  InputSameDT=on
  ffMeas : Lookup_n-D  NumberOfTableDimensions=1  BreakpointsForDimension1=sim.signals.PIDY.Time  Table=sim.signals.PIDY.FF  InternalRulePriority=Speed  RndMeth=Simplest  InputSameDT=on
  iMeas : Lookup_n-D  NumberOfTableDimensions=1  BreakpointsForDimension1=sim.signals.PIDY.Time  Table=sim.signals.PIDY.I  InternalRulePriority=Speed  RndMeth=Simplest  InputSameDT=on
  ilimMeas : Lookup_n-D  NumberOfTableDimensions=1  BreakpointsForDimension1=sim.signals.PIDY.Time  Table=sim.signals.PIDY.ILimit  InternalRulePriority=Speed  RndMeth=Simplest  InputSameDT=on
  k_FF : Constant  Value=sim.param.PIDY.FF
  kd : Constant  Value=sim.param.PIDY.D
  ki : Constant  Value=sim.param.PIDY.I
  kp : Constant  Value=sim.param.PIDY.P
  pMeas : Lookup_n-D  NumberOfTableDimensions=1  BreakpointsForDimension1=sim.signals.PIDY.Time  Table=sim.signals.PIDY.P  InternalRulePriority=Speed  RndMeth=Simplest  InputSameDT=on
  srMeas : Lookup_n-D  NumberOfTableDimensions=1  BreakpointsForDimension1=sim.signals.PIDY.Time  Table=sim.signals.PIDY.SRate  InternalRulePriority=Speed  RndMeth=Simplest  InputSameDT=on
  tarMeas : Lookup_n-D  NumberOfTableDimensions=1  BreakpointsForDimension1=sim.signals.PIDY.Time  Table=sim.signals.PIDY.Tar  InternalRulePriority=Speed  RndMeth=Simplest  InputSameDT=on
  totMeas : Lookup_n-D  NumberOfTableDimensions=1  BreakpointsForDimension1=sim.signals.RATE.Time  Table=sim.signals.RATE.YOut  InternalRulePriority=Speed  RndMeth=Simplest  InputSameDT=on
  yawRateCtrlOut : Outport
  wires:
  RAT_FLTD/1(y) -> D/2
  Sum1/1 -> Sum2/2
  RAT_FLTE/1(y) -> P/2, Calc Derivative/1(e), I/1(e)  "yawRateErr"
  limitFlg/1 -> I/2(limit_flg)
  P/1 -> Unit Delay/1, Sum1/1  "yawRateP"
  Calc Derivative/1(derivative) -> RAT_FLTD/1(u)
  Sum/1 -> Zero-Order Hold/1
  D/1 -> Unit Delay1/1, Sum1/2  "yawRateD"
  I/1(integrator) -> Sum1/3  "yawRateI"
  FF/1 -> Sum3/1  "yawRateFF"
  Sum2/1 -> Sum3/2  "yawRateTot"
  Sum3/1 -> yawRateCtrlOut/1
  RAT_FLTT/1(y) -> FF/2, Sum/1  "yawRateTarFilt"
  yawRateTar/1 -> RAT_FLTT/1(u)
  yawRateAct/1 -> Sum/2
  Zero-Order Hold/1 -> RAT_FLTE/1(u)
  k_FF/1 -> [k_FF]
  kp/1 -> [kp]
  kd/1 -> [kd]
  ki/1 -> [ki]
  Integrator maximum/1 -> [i_max]
  Cutoff Frequency FLTD/1 -> [fltd_f]
  Cutoff Frequency FLTE/1 -> [flte_f]
  Cutoff Frequency FLTT/1 -> [fltt_f]
  [k_FF] -> FF/1
  [kp] -> P/1
  [ki] -> I/3(ki)
  [i_max] -> I/4(i_max)
  [kd] -> D/3
  [fltd_f] -> RAT_FLTD/2(cutoff_freq)
  [flte_f] -> RAT_FLTE/2(cutoff_freq)
  [fltt_f] -> RAT_FLTT/2(cutoff_freq)
  pMeas/1 -> Terminator/1  "yawRatePMeas"
  iMeas/1 -> Terminator1/1  "yawRateIMeas"
  dMeas/1 -> Terminator2/1  "yawRateDMeas"
  totMeas/1 -> Terminator4/1  "yawRateTotMeas"
  tarMeas/1 -> Terminator5/1  "yawRateTarMeas"
  errMeas/1 -> Terminator3/1  "yawRateErrMeas"
  Unit Delay2/1 -> Sum2/1  "sid_axis_12"
  Slew Rate Filter Cutoff Frequency/1 -> [sr_flt_f]
  Slew Rate Maximum/1 -> [sr_max]
  Slew Rate Tau/1 -> [sr_tau]
  dmodMeas/1 -> Terminator6/1  "yawRateDmodMeas"
  srMeas/1 -> Terminator7/1  "yawRateSrMeas"
  ffMeas/1 -> Terminator8/1  "yawRateFFMeas"
  Slew Limiter/1(Dmod) -> D/1, P/3  "yawRateDmod"
  Unit Delay/1 -> Slew Limiter/1(p_out)
  Unit Delay1/1 -> Slew Limiter/6(d_out)
  [sr_max] -> Slew Limiter/2(sr_max)
  [sr_tau] -> Slew Limiter/3(sr_tau)
  [sr_flt_f] -> Slew Limiter/4(sr_flt_f)
  ilimMeas/1 -> Terminator9/1  "yawRateILimMeas"
  clkDmod/1 -> Slew Limiter/5(clock)
  chirp/1 -> Unit Delay2/1
  Clock/1 -> ilimMeas/1, tarMeas/1, totMeas/1, errMeas/1, ffMeas/1, srMeas/1, dmodMeas/1, dMeas/1, iMeas/1, pMeas/1

== system arducopter/Throttle/Input Handler ==
  note: Input Handler
      | Determines source of the inputs to the subsystem, which can
      | be either the real flight data or simulated data.
  inMeas : Inport
  inSim : Inport  Port=2
  thrMan : Inport  Port=3
  Bus Creator : BusCreator  Inputs=9
  Bus Selector : BusSelector  OutputSignals=throttle.thrIn
  Bus Selector1 : BusSelector  OutputSignals=CTUN.thrInMeas,CTUN.angBst,BAT.batRestVoltEst,BAT.batCurr,BAT.batRes,BAT.batVolt,BARO.baroAlt,BARO.baroAirPress,BARO.baroGndTemp
  Switch : Switch  Criteria=u2 > Threshold
  data_in : Outport
  wires:
  inSim/1 -> Bus Selector/1
  inMeas/1 -> Bus Selector1/1
  thrMan/1 -> Switch/2
  Bus Selector/1 -> Switch/3  "<thrIn>"
  Bus Selector1/1 -> Switch/1  "<thrInMeas>"
  Bus Selector1/9 -> Bus Creator/9  "<baroGndTemp>"
  Bus Selector1/8 -> Bus Creator/8  "<baroAirPress>"
  Bus Selector1/7 -> Bus Creator/7  "<baroAlt>"
  Bus Selector1/6 -> Bus Creator/6  "<batVolt>"
  Bus Selector1/5 -> Bus Creator/5  "<batRes>"
  Bus Selector1/4 -> Bus Creator/4  "<batCurr>"
  Bus Selector1/3 -> Bus Creator/3  "<batRestVoltEst>"
  Bus Selector1/2 -> Bus Creator/2  "<angBst>"
  Switch/1 -> Bus Creator/1  "thrTar"
  Bus Creator/1 -> data_in/1

== system arducopter/Throttle/Throttle Calculations ==
  note: Throttle Calculations.
  note: This subsystem calculates the relevant quantities for the following throttle mixing.
      | This subsystem is mainly based on AC_AttitudeControl_Multi.cpp and AC_MotorsMulticopter.cpp.
  thrIn : Inport
  angBst : Inport  Port=2
  batRestVoltEst : Inport  Port=3
  batCurr : Inport  Port=4
  batRes : Inport  Port=5
  batVolt : Inport  Port=6
  baroAlt : Inport  Port=7
  baroAirPress : Inport  Port=8
  baroGndTemp : Inport  Port=9
  zVelCtrlRatio : Inport  Port=10
  zVelDes : Inport  Port=11
  zVelAct : Inport  Port=12
  thrMan : Inport  Port=13
  Air density Calculation : Subsystem
  Boost and Premixing : Subsystem  TreatAsAtomicUnit=on  SystemSampleTime=sim.param.dt
  Get compensation gain : MATLAB Function  TreatAsAtomicUnit=on
  Lowpass Filter : Subsystem
  Terminator1 : Terminator
  Throttle Hover : Subsystem  TreatAsAtomicUnit=on  SystemSampleTime=0.1
  Throttle Limiting based on battery state : Subsystem
  Throttle-Attitude-Mixing : Subsystem
  Unit Delay2 : UnitDelay  InitialCondition=sim.init.CTUN.ThrOut  SampleTime=-1  HasFrameUpgradeWarning=on
  thrOutFilt : Outport
  thrAvgMax : Outport  Port=2
  thrThstMax : Outport  Port=3
  comp_gain : Outport  Port=4
  thrHover : Outport  Port=5
  wires:
  Throttle Hover/1(thrHover) -> [thrHover]
  Get compensation gain/1(compGain) -> comp_gain/1  "compGain"
  Throttle Limiting based on battery state/1(liftMax) -> Get compensation gain/1(liftMax)  "liftMax"
  [thrFilt] -> Unit Delay2/1
  Throttle Limiting based on battery state/2(batVoltRestEstAct) -> Terminator1/1
  [thrHover] -> Throttle Limiting based on battery state/5(thrHover)
  Unit Delay2/1 -> Throttle Hover/3(thrAct)
  Throttle Limiting based on battery state/3(thrThstMax) -> thrThstMax/1  "thrThstMax"
  [thrFilt] -> thrOutFilt/1
  Lowpass Filter/1(thrOutFilt) -> [thrFilt]
  angBst/1 -> Boost and Premixing/4(angBst)
  [thrHover] -> Boost and Premixing/3(thrHover)
  Boost and Premixing/2(thrAvgMax) -> thrAvgMax/1
  batRestVoltEst/1 -> Throttle Limiting based on battery state/1(batRestVoltEst)
  batCurr/1 -> Throttle Limiting based on battery state/2(batCurr)
  batRes/1 -> Throttle Limiting based on battery state/3(batRes)
  batVolt/1 -> Throttle Limiting based on battery state/4(batVolt)
  baroAlt/1 -> Air density Calculation/1(baroAlt)
  baroAirPress/1 -> Air density Calculation/2(baroAirPress)
  baroGndTemp/1 -> Air density Calculation/3(baroGndTemp)
  Boost and Premixing/1(thrOutRaw) -> Lowpass Filter/1(thrOutRaw)
  [thrHover] -> thrHover/1
  [thrIn] -> Boost and Premixing/2(thrIn)
  thrIn/1 -> [thrIn]
  zVelCtrlRatio/1 -> Throttle-Attitude-Mixing/2(zVelCtrlRatio)
  thrMan/1 -> Throttle-Attitude-Mixing/4(thrMan)
  Throttle-Attitude-Mixing/1(thrRPYMix) -> Boost and Premixing/1(thrRPYMix)
  [thrIn] -> Throttle-Attitude-Mixing/1(thrIn)
  zVelDes/1 -> [zVelDes]
  [zVelDes] -> Throttle-Attitude-Mixing/3(zVelDes)
  [zVelDes] -> Throttle Hover/2(zVelDes)
  zVelAct/1 -> Throttle Hover/1(zVelAct)
  Air density Calculation/1(airDensityRatio) -> Get compensation gain/2(airDensityRatio)  "airDensityRatio"

== system arducopter/Attitude Controller/input_euler_angle_roll_pitch_euler_rate_yaw()/Add feedforward to angVelBody ==
  note: Thrust error angle above which yaw corrections are limited
  angVelBodyFeedforward : Inport
  angVelBodyIn : Inport  Port=2
  thurstErrorAngle : Inport  Port=3
  yawRateAct : Inport  Port=4
  Constant : Constant  Value=sim.param.ATC.THRUST_ERROR_ANGLE
  MATLAB Function : MATLAB Function  TreatAsAtomicUnit=on
  angVelBody : Outport
  feedforwardScaler : Outport  Port=2
  wires:
  angVelBodyFeedforward/1 -> MATLAB Function/1(angVelBodyFeedforward)
  angVelBodyIn/1 -> MATLAB Function/2(angVelBodyIn)
  thurstErrorAngle/1 -> MATLAB Function/3(thrustErrorAngle)
  yawRateAct/1 -> MATLAB Function/4(yawRateAct)
  MATLAB Function/1(angVelBodyNew) -> angVelBody/1
  Constant/1 -> MATLAB Function/5(maxThrustErrorAngle4YawCorr)
  MATLAB Function/2(feedforwardScaler) -> feedforwardScaler/1

== system arducopter/Attitude Controller/input_euler_angle_roll_pitch_euler_rate_yaw()/Feedforward disabled ==
  note: QuaternionT<T>::from_euler()
      | Computes the quaternion from the given euler angles
  note: This subsystem represents to part of input_euler_angle_roll_pitch_euler_rate_yaw() that is executed, when the feedforward is disabled ( ATC_RATE_FF_ENAB = 0 )
  eulerAngleTar : Inport
  eulerInputDes : Inport  Port=2
  Constant : Constant  Value=0  OutDataTypeStr=single
  Constant1 : Constant  Value=0  OutDataTypeStr=single
  Demux : Demux  Outputs=3
  Gain : Gain  Gain=sim.param.dt
  MATLAB Function : MATLAB Function  TreatAsAtomicUnit=on
  Selector : Selector  InputPortWidth=3  IndexOptions=Index vector (dialog)  Indices=[3]  OutputSizes=1
  Sum : Sum  Inputs=|++
  eulerRateTar : Outport
  angVelTar : Outport  Port=2
  attitudeTarget : Outport  Port=3
  wires:
  MATLAB Function/1(q) -> attitudeTarget/1  "attitudeTarget"
  Demux/1 -> MATLAB Function/1(roll)
  Demux/2 -> MATLAB Function/2(pitch)
  eulerInputDes/1 -> Demux/1
  Demux/3 -> Gain/1
  Gain/1 -> Sum/1
  Sum/1 -> MATLAB Function/3(yaw)
  eulerAngleTar/1 -> Selector/1
  Constant/1 -> eulerRateTar/1
  Constant1/1 -> angVelTar/1
  Selector/1 -> Sum/2

== system arducopter/Attitude Controller/input_euler_angle_roll_pitch_euler_rate_yaw()/Feedforward enabled ==
  note: euler_rate_to_ang_vel()
      | Converts the target euler rates into a target frame angular velocity vector for feedforward
  note: euler_accel_limit()
      | Translation of acceleration limits eulerAccelMax to the body frame
  note: This subsystem represents to part of input_euler_angle_roll_pitch_euler_rate_yaw() that is executed, when the feedforward is enabled (ATC_RATE_FF_ENAB = 1)
  note: Maximum angular accelerations in earth frame
  note: Input shaping
      | Computes target euler rates based on the error between latest angle target and the desired angle by the pilot, thereby considering acceleration limits.
  note: ang_vel_limit()
      | Ensures that angular velocites do not go over configured rate limits
  note: ang_vel_to_euler_rate()
      | Converts the target body-frame angular velocites into target euler rates
  eulerRateTarIn : Inport
  eulerAngleTar : Inport  Port=2
  eulerInputDes : Inport  Port=3
  Constant : Constant  Value=sim.param.ATC.ACCEL_R_MAX
  Constant1 : Constant  Value=sim.param.ATC.ACCEL_P_MAX
  Constant2 : Constant  Value=sim.param.ATC.ACCEL_Y_MAX
  Constant3 : Constant  Value=sim.param.ATC.RATE_R_MAX
  Constant4 : Constant  Value=sim.param.ATC.RATE_P_MAX
  Constant5 : Constant  Value=sim.param.ATC.RATE_Y_MAX
  Gain : Gain  Gain=pi/180
  Gain1 : Gain  Gain=pi/180
  Gain2 : Gain  Gain=pi/180
  MATLAB Function : MATLAB Function  TreatAsAtomicUnit=on
  MATLAB Function1 : MATLAB Function  TreatAsAtomicUnit=on
  MATLAB Function2 : MATLAB Function  TreatAsAtomicUnit=on
  MATLAB Function3 : MATLAB Function  TreatAsAtomicUnit=on
  Mux : Mux  Inputs=3
  cdeg/ss to rad/ss : Gain  Gain=0.01*pi/180
  input shaping : Subsystem
  eulerRateTarOut : Outport
  angVelTar : Outport  Port=2
  wires:
  [eulerAngleTar] -> MATLAB Function/1(eulerAngleTar), MATLAB Function1/1(eulerAngle), input shaping/1(eulerAngleTar)
  Constant/1 -> Mux/1
  Mux/1 -> cdeg/ss to rad/ss/1
  Constant1/1 -> Mux/2
  Constant2/1 -> Mux/3
  MATLAB Function/1(eulerAccelMaxBF) -> input shaping/4(eulerAccelMax)
  eulerInputDes/1 -> input shaping/2(eulerInputDes)
  eulerRateTarIn/1 -> input shaping/3(eulerRateTarIn)
  input shaping/1(eulerRateTar) -> MATLAB Function1/2(eulerRate)  "eulerRateTar"
  MATLAB Function1/1(angVelTar) -> MATLAB Function2/1(angVelTar)  "angVelTar"
  Gain/1 -> MATLAB Function2/2(angVelRollMax)
  Constant3/1 -> Gain/1
  Constant4/1 -> Gain1/1
  Gain1/1 -> MATLAB Function2/3(angVelPitchMax)
  Gain2/1 -> MATLAB Function2/4(angVelYawMax)
  Constant5/1 -> Gain2/1
  eulerAngleTar/1 -> [eulerAngleTar]  "eulerAngleTar"
  [eulerAngleTar] -> MATLAB Function3/2(eulerAngle)
  MATLAB Function3/1(eulerRate) -> eulerRateTarOut/1
  MATLAB Function2/1(angVelTarLimited) -> [angVelTar]
  [angVelTar] -> MATLAB Function3/1(angVelBf)
  [angVelTar] -> angVelTar/1
  cdeg/ss to rad/ss/1 -> MATLAB Function/2(eulerAccelMaxEF)

== system arducopter/Attitude Controller/input_euler_angle_roll_pitch_euler_rate_yaw()/Update attitudeTarget ==
  note: Normalize attitudeTarget
  note: Use angVelTar to rotate attitudeTarget
  note: Use rotated attitudeTarget, if FF is enabled.
      | Otherwise, use unchanged attitudeTarget
  attitudeTarget : Inport
  angVelTar : Inport  Port=2
  ffEnabled : Inport  Port=3
  MATLAB Function : MATLAB Function  TreatAsAtomicUnit=on
  Rotate target attitude : Subsystem
  Switch : Switch  Criteria=u2 > Threshold
  attitudeTargetUpdate : Outport
  wires:
  MATLAB Function/1(qNorm) -> attitudeTargetUpdate/1
  Switch/1 -> MATLAB Function/1(q)
  ffEnabled/1 -> Switch/2
  attitudeTarget/1 -> Switch/3, Rotate target attitude/1(attitudeTarget)
  angVelTar/1 -> Rotate target attitude/2(angVelTar)
  Rotate target attitude/1(attitudeTargetRot) -> Switch/1

== system arducopter/Attitude Controller/input_euler_angle_roll_pitch_euler_rate_yaw()/reset yaw targets ==
  note: "ahrs.yaw - euler_angle_target.z"
  note: This subsystem resets the yaw target angle and rate, if the throttle is zero, meaning that the copter is landed. The respective function is AC_AttitudeControl::reset_yaw_target_and_rate() , which is called in ModeStabilize::run() when the copter is armed, but throttle is still zero.
  eulerRateTarIn : Inport
  attitudeTargetIn : Inport  Port=2
  eulerAngleAct : Inport  Port=3
  throttle : Inport  Port=4
  Demux : Demux  Outputs=3
  Demux1 : Demux  Outputs=3
  MATLAB Function1 : MATLAB Function  TreatAsAtomicUnit=on
  MATLAB Function5 : MATLAB Function  TreatAsAtomicUnit=on
  MATLAB Function9 : MATLAB Function  TreatAsAtomicUnit=on
  Mux : Mux  Inputs=3
  Mux1 : Mux  Inputs=3
  Subtract : Sum  Inputs=-+
  Switch : Switch  Criteria=u2 > Threshold
  Switch1 : Switch  Criteria=u2 > Threshold
  Terminator{,1..4} (5 alike) : Terminator
  Zero : Constant  Value=0  OutDataTypeStr=single
  Zero1 : Constant  Value=0  OutDataTypeStr=single
  Zero2 : Constant  Value=0  OutDataTypeStr=single
  eulerRateTar : Outport
  attitudeTarget : Outport  Port=2
  wires:
  Switch1/1 -> attitudeTarget/1
  Switch/1 -> eulerRateTar/1
  throttle/1 -> Switch1/2, Switch/2
  eulerRateTarIn/1 -> Demux1/1, Switch/1
  eulerAngleAct/1 -> Demux/1
  MATLAB Function9/1(qRes) -> Switch1/3
  attitudeTargetIn/1 -> Switch1/1, MATLAB Function9/2(q2), MATLAB Function1/1(q)
  MATLAB Function1/3(yaw) -> Subtract/1  "yawAngleTar"
  MATLAB Function1/1(roll) -> Terminator/1
  MATLAB Function1/2(pitch) -> Terminator1/1
  Demux/1 -> Terminator2/1
  Demux/2 -> Terminator3/1
  Demux/3 -> Subtract/2
  Subtract/1 -> Mux/3
  MATLAB Function5/1(q) -> MATLAB Function9/1(q1)  "attitudeTargetUpdate"
  Mux/1 -> MATLAB Function5/1(vec)
  Zero/1 -> Mux/1
  Zero1/1 -> Mux/2
  Mux1/1 -> Switch/3
  Demux1/1 -> Mux1/1
  Demux1/2 -> Mux1/2
  Demux1/3 -> Terminator4/1
  Zero2/1 -> Mux1/3

== system arducopter/Attitude Controller/input_euler_angle_roll_pitch_euler_rate_yaw()/thrust_heading_rotation_angles() ==
  note: Limit yaw error based in maximum acceleration
  note: AC_AttitudeControl::thrust_vector_rotation_angles()
      | Calculation of thrust_angle, thrust_error_angle, attitude_error and thrust_vector_correction
  note: This subsystem contains all the calculations contained in the function AC_AttitudeControl::thrust_heading_rotation_angles() that is called in AC_AttitudeControl::attitude_controller_run_quat()
  attitudeTargetIn : Inport
  attitudeBodyAct : Inport  Port=2
  Yaw error limitation : Subsystem
  thrust_vector_rotation_angles() : Subsystem
  attitudeTarget : Outport
  attitudeError : Outport  Port=2
  thrustErrorAngle : Outport  Port=3
  thrustAngle : Outport  Port=4
  wires:
  attitudeTargetIn/1 -> [attitudeTarget]  "attTar"
  [attitudeBody] -> thrust_vector_rotation_angles()/2(attitudeBodyAct)
  thrust_vector_rotation_angles()/1(attitudeError) -> Yaw error limitation/1(attitudeErrorIn)
  thrust_vector_rotation_angles()/3(thrustErrAngle) -> thrustErrorAngle/1
  thrust_vector_rotation_angles()/2(thrustVecCorrection) -> Yaw error limitation/2(thrustVecCorrection)
  thrust_vector_rotation_angles()/4(thrustAngle) -> thrustAngle/1
  attitudeBodyAct/1 -> [attitudeBody]  "attBody"
  [attitudeBody] -> Yaw error limitation/3(attitudeBody)
  Yaw error limitation/1(atitudeTarget) -> attitudeTarget/1
  Yaw error limitation/2(attitudeError) -> attitudeError/1
  [attitudeTarget] -> thrust_vector_rotation_angles()/1(attitudeTarget)
  [attitudeTarget] -> Yaw error limitation/4(attitudeTarget)
